simulink library "dsppolyfun"  (Simulink 5.0)
undefined symbols (not defined in the file or in its folder): V
libraries: dspsolvers x1
settings Model: RequirementInfo=9  CovMetricSettings=d  Creator=sconahan  LastModifiedBy=mkhan  TargetHWChar=2  TargetHWWordLengths=8,16,32,32

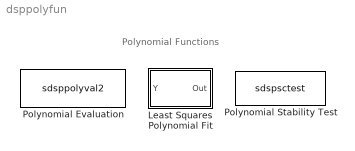
== system dsppolyfun ==
  note: Polynomial Functions
  Least Squares Polynomial Fit : Subsystem  mask(Least Squares Polynomial Fit){X=(0:31) / 31, N=3}
      mask prompts: X "Control points (X):"; N "Polynomial order (N):"
      mask help: Find the coefficients of a polynomial P(X) of order N that fits the input data U, such that P(X) best approximates U in a least-squares sense. The input vector U must have the same length as X.
      mask init:
      | % construct Vandermonde matrix
      | X=X(:); V(:,N+1) = ones(length(X),1); V(:,N) = X;
      | for j = N-1:-1:1, V(:,j) = X.*V(:,j+1); end
      mask Help: web(dspbhelp);
      mask Display: disp('Polyfit')
  Polynomial Evaluation : S-Function  FunctionName=sdsppolyval2  Parameters=constCoeffs,useConstCoeffs  mask(Polynomial Evaluation){useConstCoeffs=off, constCoeffs=[5 4 3 2 1]}
      mask prompts: useConstCoeffs "Use constant coefficients"; constCoeffs "Constant coefficients:"
      mask help:
      | Apply specified polynomial function to input.
      |
      | Example: [1 3 5] represents u^2 + 3u + 5.
      mask init:
      | [p,xy] = dspblkpolyval('icon');
      mask Help: web(dspbhelp);
      mask CallbackString: dspblkpolyval|
      mask Display:
      | port_label(p.in1,   p.i1,  p.i1s);
      | port_label(p.in2,   p.i2,  p.i2s);
      | port_label(p.out, p.o1, p.o1s);
      | disp('Polyval')
  Polynomial Stability Test : S-Function  FunctionName=sdspsctest
      mask Type: Polynomial Stability Test
      mask Description: Determines if all roots of the input polynomial lie inside the unit circle.  Implemented using the Schur-Cohn algorithm.
      mask Help: web(dspbhelp);
      mask Display: disp('|roots(u)| < 1')

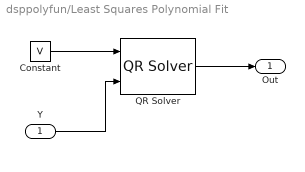
== system dsppolyfun/Least Squares Polynomial Fit ==
  Y : Inport
  Constant : Constant  Value=V
  QR Solver : dspsolvers/QR Solver
  Out : Outport
  wires:
  Y/1 -> QR Solver/2
  QR Solver/1 -> Out/1
  Constant/1 -> QR Solver/1
